simulink model "mbk"  (R2020a)
settings: Solver=ode4  StartTime=0.0  StopTime=50  FixedStep=0.01  RelTol=1e-3
InitFcn:
  | MBK
undefined symbols (not defined in the file): b, k, m
settings Model: Creator=Ali  LastModifiedBy=Ali
settings DataIOCC: ReturnWorkspaceOutputs=off
settings DebuggingCC: ArithmeticOperatorsInVariantConditions=warning
settings SFSimCC: SimUseLocalCustomCode=off  CustomCodeUndefinedFunction=UseInterfaceOnly
settings RTWCC: RTWUseLocalCustomCode=off

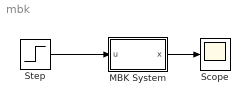
== system mbk ==
  MBK System : Subsystem
  Scope : Scope
  Step : Step  SampleTime=0
  wires:
  MBK System/1(x) -> Scope/1
  Step/1 -> MBK System/1(u)

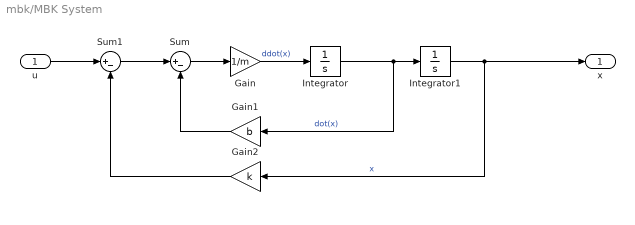
== system mbk/MBK System ==
  u : Inport
  Gain : Gain  Gain=1/m
  Gain1 : Gain  Gain=b
  Gain2 : Gain  Gain=k
  Integrator : Integrator
  Integrator1 : Integrator
  Sum : Sum  Inputs=|+-
  Sum1 : Sum  Inputs=|+-
  x : Outport
  wires:
  Gain2/1 -> Sum1/2
  Gain/1 -> Integrator/1  "ddot(x)"
  Integrator/1 -> Gain1/1, Integrator1/1  "dot(x)"
  u/1 -> Sum1/1
  Sum/1 -> Gain/1
  Gain1/1 -> Sum/2
  Integrator1/1 -> x/1, Gain2/1  "x"
  Sum1/1 -> Sum/1
